simulink model "test_steamjacket"  (R2021b)
settings: Solver=VariableStepAuto  StartTime=0.0  StopTime=10.0  RelTol=1e-3
settings Model: Creator=Edwar  LastModifiedBy=Edwar

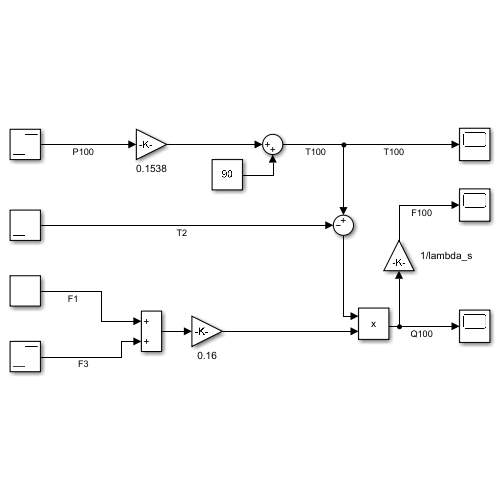
[thumbnail: Simulink's stored preview of the top-level diagram]
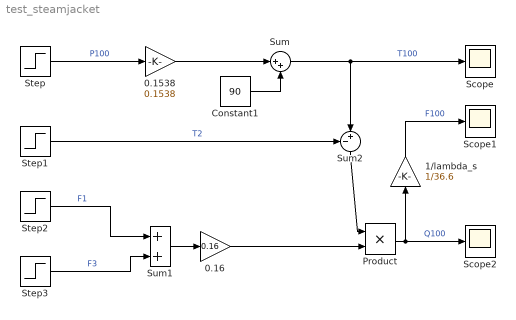
== system test_steamjacket ==
  0.1538 : Gain  Gain=0.1538
  0.16 : Gain  Gain=0.16
  1/lambda_s : Gain  Gain=1/36.6
  Constant1 : Constant  Value=90
  Product : Product
  Scope : Scope
  Scope1 : Scope
  Scope2 : Scope
  Step : Step  SampleTime=0
  Step1 : Step  Time=3  SampleTime=0
  Step2 : Step  Time=2  SampleTime=0
  Step3 : Step  Time=4  SampleTime=0
  Sum : Sum  Inputs=|++
  Sum1 : Sum
  Sum2 : Sum  Inputs=-+|
  wires:
  Step/1 -> 0.1538/1  "P100"
  0.1538/1 -> Sum/1
  Constant1/1 -> Sum/2
  Sum/1 -> Scope/1, Sum2/2  "T100"
  Step2/1 -> Sum1/1  "F1"
  Step3/1 -> Sum1/2  "F3"
  Sum1/1 -> 0.16/1
  Step1/1 -> Sum2/1  "T2"
  Sum2/1 -> Product/1
  0.16/1 -> Product/2
  Product/1 -> Scope2/1, 1/lambda_s/1  "Q100"
  1/lambda_s/1 -> Scope1/1  "F100"
